simulink model "Adaptation_To_C_Code"  (R2018b)
settings: Solver=ode4  StartTime=0.0  StopTime=10.0  FixedStep=0.002  RelTol=1e-3
undefined symbols (not defined in the file): delta_negative_l, delta_negative_r, delta_positive_l, delta_positive_r, DiscIntNeverNeededParam, kd_l, kd_r, ki_l, ki_r, kp_l, kp_r
libraries: simulink x2
settings Model: Creator=Pedro Saman  LastModifiedBy=Pedro Saman

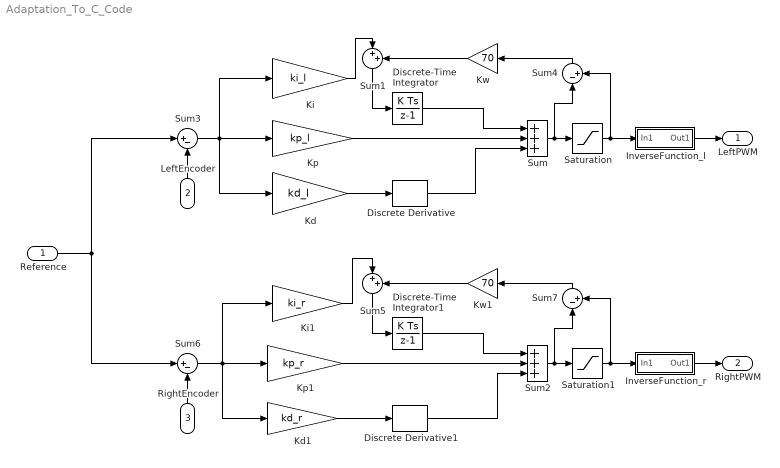
== system Adaptation_To_C_Code ==
  "Reference " : Inport
  "LeftEncoder " : Inport  Port=2
  "RightEncoder " : Inport  Port=3
  Discrete Derivative : simulink/Discrete/Discrete Derivative  gainval=1.0  ICPrevScaledInput=0.0  OutMin=[]  OutMax=[]  OutDataType=fixdt(1, 16)  OutScaling=2^-10  DoSatur=off
  Discrete Derivative1 : simulink/Discrete/Discrete Derivative  gainval=1.0  ICPrevScaledInput=0.0  OutMin=[]  OutMax=[]  OutDataType=fixdt(1, 16)  OutScaling=2^-10  DoSatur=off
  Discrete-Time Integrator : DiscreteIntegrator  SampleTime=-1  ICPrevOutput=DiscIntNeverNeededParam  ICPrevScaledInput=DiscIntNeverNeededParam
  Discrete-Time Integrator1 : DiscreteIntegrator  SampleTime=-1  ICPrevOutput=DiscIntNeverNeededParam  ICPrevScaledInput=DiscIntNeverNeededParam
  "InverseFunction_l " : Subsystem
  "InverseFunction_r " : Subsystem
  Kd : Gain  Gain=kd_l
  Kd1 : Gain  Gain=kd_r
  Ki : Gain  Gain=ki_l
  Ki1 : Gain  Gain=ki_r
  Kp : Gain  Gain=kp_l
  Kp1 : Gain  Gain=kp_r
  Kw : Gain  Gain=70
  Kw1 : Gain  Gain=70
  Saturation : Saturate  UpperLimit=255  LowerLimit=-255
  Saturation1 : Saturate  UpperLimit=255  LowerLimit=-255
  Sum : Sum  Inputs=|+|+|+|
  Sum1 : Sum  Inputs=|++
  Sum2 : Sum  Inputs=|+|+|+|
  Sum3 : Sum  Inputs=|+-
  Sum4 : Sum  Inputs=|-+
  Sum5 : Sum  Inputs=|++
  Sum6 : Sum  Inputs=|+-
  Sum7 : Sum  Inputs=|-+
  "LeftPWM " : Outport
  RightPWM : Outport  Port=2
  wires:
  Kw/1 -> Sum1/2
  Ki/1 -> Sum1/1
  Sum4/1 -> Kw/1
  "RightEncoder "/1 -> Sum6/2
  Ki1/1 -> Sum5/1
  "InverseFunction_r "/1(Out1) -> RightPWM/1
  Discrete-Time Integrator/1 -> Sum/1
  Kd/1 -> Discrete Derivative/1
  Kd1/1 -> Discrete Derivative1/1
  Sum1/1 -> Discrete-Time Integrator/1
  Sum7/1 -> Kw1/1
  Discrete Derivative/1 -> Sum/3
  Kw1/1 -> Sum5/2
  "InverseFunction_l "/1(Out1) -> "LeftPWM "/1
  "Reference "/1 -> Sum6/1, Sum3/1
  Sum/1 -> Sum4/1, Saturation/1
  Sum5/1 -> Discrete-Time Integrator1/1
  Kp1/1 -> Sum2/2
  "LeftEncoder "/1 -> Sum3/2
  Sum3/1 -> Kd/1, Ki/1, Kp/1
  Discrete-Time Integrator1/1 -> Sum2/1
  Sum2/1 -> Sum7/1, Saturation1/1
  Saturation1/1 -> "InverseFunction_r "/1(In1), Sum7/2
  Kp/1 -> Sum/2
  Saturation/1 -> "InverseFunction_l "/1(In1), Sum4/2
  Discrete Derivative1/1 -> Sum2/3
  Sum6/1 -> Kd1/1, Ki1/1, Kp1/1

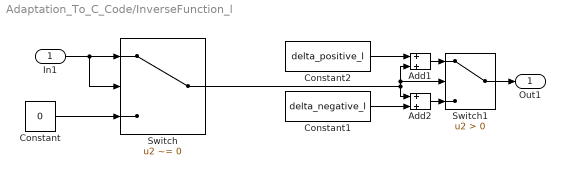
== system Adaptation_To_C_Code/InverseFunction_l  ==
  In1 : Inport
  Add1 : Sum
  Add2 : Sum
  Constant : Constant  Value=0
  Constant1 : Constant  Value=delta_negative_l
  Constant2 : Constant  Value=delta_positive_l
  Switch : Switch  Criteria=u2 ~= 0
  Switch1 : Switch  Criteria=u2 > Threshold
  Out1 : Outport
  wires:
  Switch/1 -> Add1/2, Switch1/2, Add2/1
  Constant1/1 -> Add2/2
  In1/1 -> Switch/2, Switch/1
  Constant/1 -> Switch/3
  Switch1/1 -> Out1/1
  Add2/1 -> Switch1/3
  Add1/1 -> Switch1/1
  Constant2/1 -> Add1/1

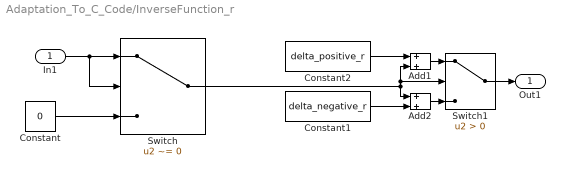
== system Adaptation_To_C_Code/InverseFunction_r  ==
  In1 : Inport
  Add1 : Sum
  Add2 : Sum
  Constant : Constant  Value=0
  Constant1 : Constant  Value=delta_negative_r
  Constant2 : Constant  Value=delta_positive_r
  Switch : Switch  Criteria=u2 ~= 0
  Switch1 : Switch  Criteria=u2 > Threshold
  Out1 : Outport
  wires:
  Switch/1 -> Add1/2, Switch1/2, Add2/1
  Constant1/1 -> Add2/2
  In1/1 -> Switch/2, Switch/1
  Constant/1 -> Switch/3
  Switch1/1 -> Out1/1
  Add2/1 -> Switch1/3
  Add1/1 -> Switch1/1
  Constant2/1 -> Add1/1
